simulink model "ConstantMem_4"  (R2021a)
settings: Solver=FixedStepAuto  StartTime=0.0  StopTime=10.0  RelTol=1e-3  EnableMultiTasking=on
settings Model: DataDictionary=worldDD.sldd  SILPILModeSetting=veronly  ExtModeTrigDuration=2  Creator=Koorosh  LastModifiedBy=Koorosh
settings OptimizationCC: EnhancedBackFolding=on  PassReuseOutputArgsAs=Individual arguments  ZeroExternalMemoryAtStartup=off  ZeroInternalMemoryAtStartup=off  MaxStackSize=64  OptimizeBlockOrder=speed  DifferentSizesBufferReuse=on  OptimizationCustomize=off  EfficientTunableParamExpr=on
settings DebuggingCC: ParameterTunabilityLossMsg=error
settings HardwareCC: ProdBitPerInt=16  ProdBitPerPointer=16  ProdBitPerSizeT=16  ProdBitPerPtrDiffT=16  ProdLargestAtomicFloat=None  ProdWordSize=8  ProdHWDeviceType=Atmel->AVR
settings SFSimCC: MATLABDynamicMemAlloc=off
settings RTWCC: SystemTargetFile=ert.tlc  HardwareBoard=Arduino Uno  TemplateMakefile=ert_default_tmf  Toolchain=Arduino AVR  BuildConfiguration=Faster Runs
settings CodeAppCC: ForceParamTrailComments=on  IgnoreCustomStorageClasses=off  OperatorAnnotations=on  SimulinkDataObjDesc=on  SFDataObjDesc=on  InsertBlockDesc=on
settings ERTTargetCC: SupportContinuousTime=on  SupportVariableSizeSignals=on  ExtModeStaticAllocSize=250

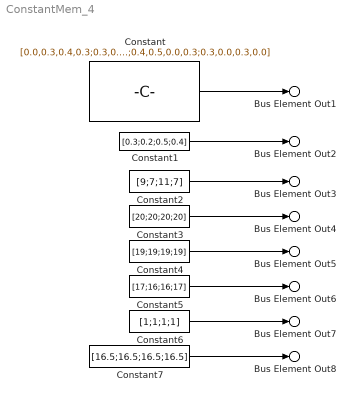
== system ConstantMem_4 ==
  Constant : Constant  Value=[0.0,0.3,0.4,0.3;0.3,0.0,0.5,0.0;0.4,0.5,0.0,0.3;0.3,0.0,0.3,0.0]
  Constant1 : Constant  Value=[0.3;0.2;0.5;0.4]
  Constant2 : Constant  Value=[9;7;11;7]
  Constant3 : Constant  Value=[20;20;20;20]
  Constant4 : Constant  Value=[19;19;19;19]
  Constant5 : Constant  Value=[17;16;16;17]
  Constant6 : Constant  Value=[1;1;1;1]
  Constant7 : Constant  Value=[16.5;16.5;16.5;16.5]
  Bus Element Out1 : Outport  PortName=C  Element=A
  Bus Element Out2 : Outport  PortName=C  Element=b
  Bus Element Out3 : Outport  PortName=C  Element=c
  Bus Element Out8 : Outport  PortName=C  Element=x0
  Bus Element Out4 : Outport  PortName=C  Element=off
  Bus Element Out5 : Outport  PortName=C  Element=on
  Bus Element Out6 : Outport  PortName=C  Element=get
  Bus Element Out7 : Outport  PortName=C  Element=diff
  wires:
  Constant/1 -> Bus Element Out1/1
  Constant1/1 -> Bus Element Out2/1
  Constant2/1 -> Bus Element Out3/1
  Constant3/1 -> Bus Element Out4/1
  Constant4/1 -> Bus Element Out5/1
  Constant5/1 -> Bus Element Out6/1
  Constant6/1 -> Bus Element Out7/1
  Constant7/1 -> Bus Element Out8/1
